simulink model "SecRwLtStZeroTrgtPosSelc"  (R2018b)
settings: Solver=FixedStepDiscrete  StartTime=0.0  StopTime=10.0  RelTol=1e-3
undefined symbols (not defined in the file or in its folder): KeSMSw6SAcsEntrySecRwLtStCushnFrtUpwdDnwdPos_Val, KeSMSw6SAcsEntrySecRwLtStCushnFrtUpwdDnwdPosMax_Val, KeSMSw6SAcsEntrySecRwLtStCushnFrtUpwdDnwdPosMin_Val, KeSMSw6SAcsMd56SecRwLtStCushnFrtUpwdDnwdPos_Val, KeSMSw6SAcsMd56SecRwLtStCushnFrtUpwdDnwdPosMax_Val, KeSMSw6SAcsMd56SecRwLtStCushnFrtUpwdDnwdPosMin_Val, KeSMSw6SRecoveryMdSecRwLtStCushnFrtUpwdDnwdPos_Val, KeSMSw6SRecoveryMdSecRwLtStCushnFrtUpwdDnwdPosMax_Val, KeSMSw6SRecoveryMdSecRwLtStCushnFrtUpwdDnwdPosMin_Val, KeSMSwAcsEntrySecRwLtStCushnFrtIUpwdDnwdPos_Val, KeSMSwAcsEntrySecRwLtStCushnFrtIUpwdDnwdPosMax_Val, KeSMSwAcsEntrySecRwLtStCushnFrtIUpwdDnwdPosMin_Val, KeSMSwAcsMd56SecRwLtStCushnFrtUpwdDnwdPos_Val, KeSMSwAcsMd56SecRwLtStCushnFrtUpwdDnwdPosMax_Val, KeSMSwAcsMd56SecRwLtStCushnFrtUpwdDnwdPosMin_Val, KeSMSwAcsMd8SecRwLtStCushnFrtUpwdDnwdPos_Val, KeSMSwAcsMd8SecRwLtStCushnFrtUpwdDnwdPosMax_Val, KeSMSwAcsMd8SecRwLtStCushnFrtUpwdDnwdPosMin_Val, KeSMSwRecoveryMdSecRwLtStCushnFrtUpwdDnwdPos_Val, KeSMSwRecoveryMdSecRwLtStCushnFrtUpwdDnwdPosMax_Val, KeSMSwRecoveryMdSecRwLtStCushnFrtUpwdDnwdPosMin_Val, KeSMSwSecRwLtStZeroEnTrig5576sBitMask_Val, KeSMSwSecRwLtStZeroEnTrig557BitMask_Val
libraries: TrgtPosSelcLib x5
settings Model: Creator=sn2xws  LastModifiedBy=sn2xws
settings Model: ModifiedHistory=|
  | 2024.7.8 V3.0.0 557模式流程V1.9
  | 2024.8.14 V3.0.1增加6s版bitmask标定
  | 2024.9.5 V3.0.2 增加Md56
  | 2024.9.16 V3.0.3 Md8 6s目标位置信号未连接到正确值（4095）
  | 2024.9.26 V3.0.4 只计算一次的目标位置创建static变量，避免丢失
settings DataIOCC: SaveFormat=StructureWithTime
settings OptimizationCC: DefaultParameterBehavior=Inlined  EnhancedBackFolding=on  PassReuseOutputArgsAs=Individual arguments  ZeroExternalMemoryAtStartup=off  ZeroInternalMemoryAtStartup=off  OptimizeBlockOrder=speed  DifferentSizesBufferReuse=on  OptimizationCustomize=off
settings DebuggingCC: ParameterTunabilityLossMsg=error
settings SFSimCC: MATLABDynamicMemAlloc=off
settings RTWCC: SystemTargetFile=autosar.tlc  GenCodeOnly=on  TemplateMakefile=ert_default_tmf  Description=AUTOSAR  GenerateReport=on  IncludeHyperlinkInReport=on  LaunchReport=on  GenerateTraceInfo=on  GenerateTraceReport=on  GenerateTraceReportSl=on  GenerateTraceReportSf=on  GenerateTraceReportEml=on
settings CodeAppCC: ForceParamTrailComments=on  IgnoreCustomStorageClasses=off  OperatorAnnotations=on  SimulinkDataObjDesc=on  SFDataObjDesc=on  InsertBlockDesc=on
settings STFCustomTargetCC: TargetLangStandard=C99 (ISO)  MultiwordLength=256  ParMdlRefBuildCompliant=on  CompOptLevelCompliant=on  IncludeMdlTerminateFcn=off  CombineOutputUpdateFcns=on  SuppressErrorStatus=on  ERTCustomFileBanners=on  SupportNonFinite=off  SupportComplex=off  SupportContinuousTime=off  SupportNonInlinedSFcns=off  RemoveResetFunc=on  MATLABClassNameForMDSCustomization=Simulink.SoftwareTarget.ERTCustomization  AutosarCompliant=on  UseToolchainInfoCompliant=on  LookupTableObjectStructAxisOrder=2,1,3,4,...  LUTObjectStructOrderEvenSpacing=Size,Table,Breakpoints  SystemTargetFile=autosar.tlc
settings ERTTargetCC: TargetLangStandard=C99 (ISO)  ConcurrentExecutionCompliant=off  IncludeMdlTerminateFcn=off  SuppressErrorStatus=on  SupportNonFinite=off  SupportComplex=off  ModelStepFunctionPrototypeControlCompliant=off  CPPClassGenCompliant=off  AutosarCompliant=on  LookupTableObjectStructAxisOrder=2,1,3,4,...  LUTObjectStructOrderEvenSpacing=Size,Table,Breakpoints  InlinedParameterPlacement=NonHierarchical  ERTCustomFileTemplate=example_file_process.tlc  ERTFilePackagingFormat=Compact

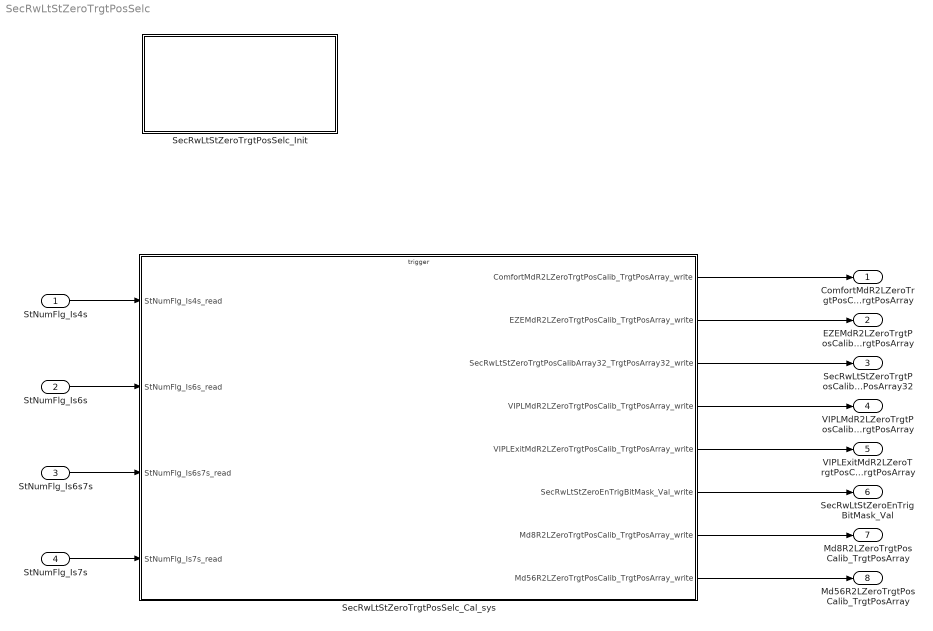
== system SecRwLtStZeroTrgtPosSelc ==
  StNumFlg_Is4s : Inport  OutDataTypeStr=boolean  PortDimensions=1
  StNumFlg_Is6s : Inport  Port=2  OutDataTypeStr=boolean  PortDimensions=1
  StNumFlg_Is6s7s : Inport  Port=3  OutDataTypeStr=boolean  PortDimensions=1
  StNumFlg_Is7s : Inport  Port=4  OutDataTypeStr=boolean  PortDimensions=1
  SecRwLtStZeroTrgtPosSelc_Cal_sys : Subsystem
  SecRwLtStZeroTrgtPosSelc_Init : Subsystem
  ComfortMdR2LZeroTrgtPosCalib_TrgtPosArray : Outport  Description=|  OutDataTypeStr=uint16  PortDimensions=3
      | 0:Pos
      | 1:Max
      | 2:Min
  EZEMdR2LZeroTrgtPosCalib_TrgtPosArray : Outport  Description=|  Port=2  OutDataTypeStr=uint16  PortDimensions=3
      | 0:Pos
      | 1:Max
      | 2:Min
  SecRwLtStZeroTrgtPosCalibArray32_TrgtPosArray32 : Outport  Description=|  Port=3  OutDataTypeStr=uint16  PortDimensions=96
      | 0:Pos
      | 1:Max
      | 2:Min
  VIPLMdR2LZeroTrgtPosCalib_TrgtPosArray : Outport  Description=|  Port=4  OutDataTypeStr=uint16  PortDimensions=3
      | 0:Pos
      | 1:Max
      | 2:Min
  VIPLExitMdR2LZeroTrgtPosCalib_TrgtPosArray : Outport  Description=|  Port=5  OutDataTypeStr=uint16  PortDimensions=3
      | 0:Pos
      | 1:Max
      | 2:Min
  SecRwLtStZeroEnTrigBitMask_Val : Outport  Port=6  OutDataTypeStr=uint32  PortDimensions=1
  Md8R2LZeroTrgtPosCalib_TrgtPosArray : Outport  Description=|  Port=7  OutDataTypeStr=uint16  PortDimensions=3
      | 0:Pos
      | 1:Max
      | 2:Min
  Md56R2LZeroTrgtPosCalib_TrgtPosArray : Outport  Description=|  Port=8  OutDataTypeStr=uint16  PortDimensions=3
      | 0:Pos
      | 1:Max
      | 2:Min
  wires:
  StNumFlg_Is4s/1 -> SecRwLtStZeroTrgtPosSelc_Cal_sys/1(StNumFlg_Is4s_read)
  StNumFlg_Is6s/1 -> SecRwLtStZeroTrgtPosSelc_Cal_sys/2(StNumFlg_Is6s_read)
  StNumFlg_Is6s7s/1 -> SecRwLtStZeroTrgtPosSelc_Cal_sys/3(StNumFlg_Is6s7s_read)
  StNumFlg_Is7s/1 -> SecRwLtStZeroTrgtPosSelc_Cal_sys/4(StNumFlg_Is7s_read)
  SecRwLtStZeroTrgtPosSelc_Cal_sys/1(ComfortMdR2LZeroTrgtPosCalib_TrgtPosArray_write) -> ComfortMdR2LZeroTrgtPosCalib_TrgtPosArray/1
  SecRwLtStZeroTrgtPosSelc_Cal_sys/2(EZEMdR2LZeroTrgtPosCalib_TrgtPosArray_write) -> EZEMdR2LZeroTrgtPosCalib_TrgtPosArray/1
  SecRwLtStZeroTrgtPosSelc_Cal_sys/3(SecRwLtStZeroTrgtPosCalibArray32_TrgtPosArray32_write) -> SecRwLtStZeroTrgtPosCalibArray32_TrgtPosArray32/1
  SecRwLtStZeroTrgtPosSelc_Cal_sys/4(VIPLMdR2LZeroTrgtPosCalib_TrgtPosArray_write) -> VIPLMdR2LZeroTrgtPosCalib_TrgtPosArray/1
  SecRwLtStZeroTrgtPosSelc_Cal_sys/5(VIPLExitMdR2LZeroTrgtPosCalib_TrgtPosArray_write) -> VIPLExitMdR2LZeroTrgtPosCalib_TrgtPosArray/1
  SecRwLtStZeroTrgtPosSelc_Cal_sys/6(SecRwLtStZeroEnTrigBitMask_Val_write) -> SecRwLtStZeroEnTrigBitMask_Val/1
  SecRwLtStZeroTrgtPosSelc_Cal_sys/7(Md8R2LZeroTrgtPosCalib_TrgtPosArray_write) -> Md8R2LZeroTrgtPosCalib_TrgtPosArray/1
  SecRwLtStZeroTrgtPosSelc_Cal_sys/8(Md56R2LZeroTrgtPosCalib_TrgtPosArray_write) -> Md56R2LZeroTrgtPosCalib_TrgtPosArray/1

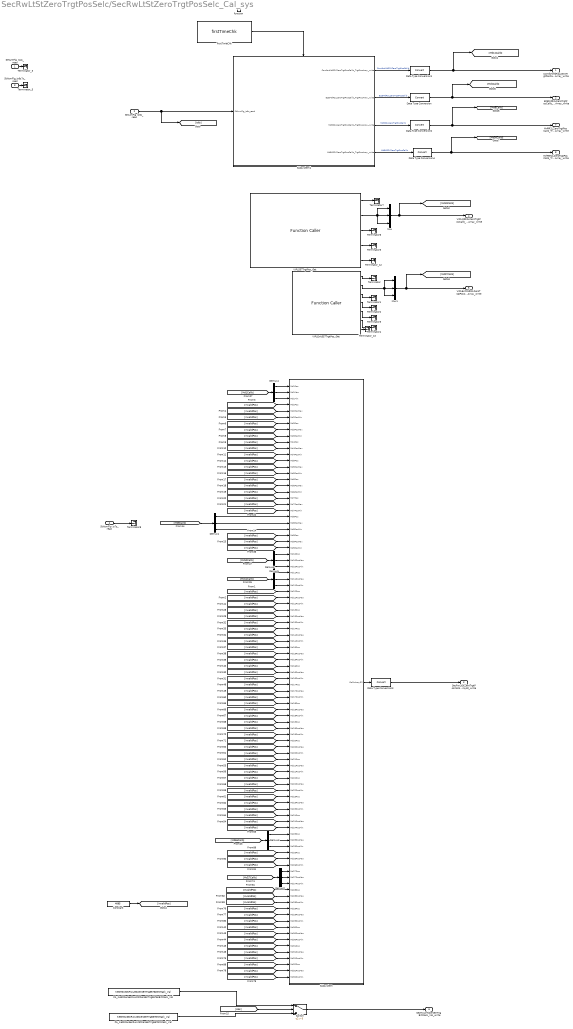
== system SecRwLtStZeroTrgtPosSelc/SecRwLtStZeroTrgtPosSelc_Cal_sys ==
  StNumFlg_Is4s_read : Inport
  StNumFlg_Is6s_read : Inport  Port=2
  StNumFlg_Is6s7s_read : Inport  Port=3
  StNumFlg_Is7s_read : Inport  Port=4
  function : TriggerPort  TriggerType=function-call  IsSimulinkFunction=on  FunctionName=SecRwLtStZeroTrgtPosSelc_Cal  VariantControl=(inherit)
  Constant : Constant  Value=4095  OutDataTypeStr=uint16
  Data Type Conversion{,1..4} (5 alike) : DataTypeConversion
  Demux{1..6} (6 alike) : Demux  Outputs=3
  Mux : Mux  Inputs=3
  Mux1 : Mux  Inputs=3
  PA_KeSMSwSecRwLtStZeroEnTrig5576sBitMask_Val : Constant  Value=KeSMSwSecRwLtStZeroEnTrig5576sBitMask_Val
  PA_KeSMSwSecRwLtStZeroEnTrig557BitMask_Val : Constant  Value=KeSMSwSecRwLtStZeroEnTrig557BitMask_Val
  Subsystem : Subsystem
  Subsystem1 : Subsystem
  Switch : Switch  Criteria=u2 > Threshold
  Terminator{,1..8} (9 alike) : Terminator
  Terminator_{3,5,12..13} (4 alike) : Terminator
  VIPL557TrgtPos_Get : FunctionCaller  FunctionPrototype=[SecRwLtStBkReclnTrgtPos,SecRwLtStZeroTrgtPos,SecRwLtStLgrstUpwdDnwdTrgtPos,SecRwLtStLgrstInwdOtwdTrgtPos,SecRwLtStFwdBkwdTrgtPos] = VIPL557TrgtPos_Get()  OutputArgumentSpecifications=uint16(1), uint16(1), uint16(1), uint16(1), uint16(1)
  VIPLExit557TrgtPos_Get : FunctionCaller  FunctionPrototype=[SecRwLtStBkReclnTrgtPos,SecRwLtStZeroTrgtPos,SecRwLtStLgrstUpwdDnwdTrgtPos,SecRwLtStLgrstInwdOtwdTrgtPos,ThdRwLtStBkReclnTrgtPos,ThdRwLtStFwdBkwdTrgtPos,SecRwLtStFwdBkwdTrgtPos] = VIPLExit557TrgtPos_Get()  OutputArgumentSpecifications=uint16(1), uint16(1), uint16(1), uint16(1), uint16(1), uint16(1), uint16(1)
  firstTimeChk : TrgtPosSelcLib/firstTimeChk  SystemSampleTime=-1
  ComfortMdR2LZeroTrgtPosCalib_TrgtPosArray_write : Outport
      settings: EnsureOutportIsVirtual=on
  EZEMdR2LZeroTrgtPosCalib_TrgtPosArray_write : Outport  Port=2
      settings: EnsureOutportIsVirtual=on
  SecRwLtStZeroTrgtPosCalibArray32_TrgtPosArray32_write : Outport  Port=3
      settings: EnsureOutportIsVirtual=on
  VIPLMdR2LZeroTrgtPosCalib_TrgtPosArray_write : Outport  Port=4
      settings: EnsureOutportIsVirtual=on
  VIPLExitMdR2LZeroTrgtPosCalib_TrgtPosArray_write : Outport  Port=5
      settings: EnsureOutportIsVirtual=on
  SecRwLtStZeroEnTrigBitMask_Val_write : Outport  Port=6
      settings: EnsureOutportIsVirtual=on
  Md8R2LZeroTrgtPosCalib_TrgtPosArray_write : Outport  Port=7
      settings: EnsureOutportIsVirtual=on
  Md56R2LZeroTrgtPosCalib_TrgtPosArray_write : Outport  Port=8
      settings: EnsureOutportIsVirtual=on
  wires:
  StNumFlg_Is4s_read/1 -> Terminator_3/1
  StNumFlg_Is6s7s_read/1 -> Terminator_5/1
  Mux/1 -> [Md10Calib], VIPLMdR2LZeroTrgtPosCalib_TrgtPosArray_write/1
  VIPLExit557TrgtPos_Get/2 -> Mux1/3, Mux1/1, Mux1/2
  Mux1/1 -> [Md27Calib], VIPLExitMdR2LZeroTrgtPosCalib_TrgtPosArray_write/1
  VIPLExit557TrgtPos_Get/1 -> Terminator/1
  VIPLExit557TrgtPos_Get/3 -> Terminator1/1
  VIPLExit557TrgtPos_Get/4 -> Terminator2/1
  VIPLExit557TrgtPos_Get/5 -> Terminator3/1
  VIPLExit557TrgtPos_Get/6 -> Terminator4/1
  VIPL557TrgtPos_Get/4 -> Terminator5/1
  VIPL557TrgtPos_Get/3 -> Terminator6/1
  VIPL557TrgtPos_Get/1 -> Terminator7/1
  VIPL557TrgtPos_Get/2 -> Mux/3, Mux/1, Mux/2
  Data Type Conversion3/1 -> SecRwLtStZeroTrgtPosCalibArray32_TrgtPosArray32_write/1
  Demux1/3 -> Subsystem/24(Md8PosMin)
  [invalidPos] -> Subsystem/85(Md29Pos)
  [invalidPos] -> Subsystem/10(Md4Pos)
  [invalidPos] -> Subsystem/17(Md6PosMax)
  [invalidPos] -> Subsystem/50(Md17PosMax)
  [invalidPos] -> Subsystem/77(Md26PosMax)
  Demux1/1 -> Subsystem/22(Md8Pos)
  [invalidPos] -> Subsystem/9(Md3PosMin)
  [invalidPos] -> Subsystem/76(Md26Pos)
  [invalidPos] -> Subsystem/25(Md9Pos)
  [invalidPos] -> Subsystem/46(Md16Pos)
  [invalidPos] -> Subsystem/72(Md24PosMin)
  Demux5/3 -> Subsystem/30(Md10PosMin)
  [invalidPos] -> Subsystem/45(Md15PosMin)
  [invalidPos] -> Subsystem/20(Md7PosMax)
  [invalidPos] -> Subsystem/63(Md21PosMin)
  [invalidPos] -> Subsystem/58(Md20Pos)
  [invalidPos] -> Subsystem/53(Md18PosMax)
  Demux4/1 -> Subsystem/1(Md1Pos)
  [invalidPos] -> Subsystem/55(Md19Pos)
  [invalidPos] -> Subsystem/86(Md29PosMax)
  [invalidPos] -> Subsystem/68(Md23PosMax)
  [invalidPos] -> Subsystem/62(Md21PosMax)
  [invalidPos] -> Subsystem/14(Md5PosMax)
  [invalidPos] -> Subsystem/87(Md29PosMin)
  Demux1/2 -> Subsystem/23(Md8PosMax)
  [invalidPos] -> Subsystem/26(Md9PosMax)
  [invalidPos] -> Subsystem/94(Md32Pos)
  [invalidPos] -> Subsystem/54(Md18PosMin)
  [invalidPos] -> Subsystem/61(Md21Pos)
  [invalidPos] -> Subsystem/5(Md2PosMax)
  [invalidPos] -> Subsystem/13(Md5Pos)
  [invalidPos] -> Subsystem/96(Md32PosMin)
  [invalidPos] -> Subsystem/59(Md20PosMax)
  [invalidPos] -> Subsystem/78(Md26PosMin)
  [invalidPos] -> Subsystem/11(Md4PosMax)
  Demux3/1 -> Subsystem/73(Md25Pos)
  [invalidPos] -> Subsystem/66(Md22PosMin)
  [invalidPos] -> Subsystem/16(Md6Pos)
  Demux4/2 -> Subsystem/2(Md1Max)
  [invalidPos] -> Subsystem/70(Md24Pos)
  [invalidPos] -> Subsystem/44(Md15PosMax)
  [invalidPos] -> Subsystem/60(Md20PosMin)
  [invalidPos] -> Subsystem/64(Md22Pos)
  [invalidPos] -> Subsystem/51(Md17PosMin)
  [invalidPos] -> Subsystem/43(Md15Pos)
  [invalidPos] -> Subsystem/57(Md19PosMin)
  [invalidPos] -> Subsystem/18(Md6PosMin)
  [invalidPos] -> Subsystem/67(Md23Pos)
  [invalidPos] -> Subsystem/4(Md2Pos)
  [invalidPos] -> Subsystem/49(Md17Pos)
  [invalidPos] -> Subsystem/71(Md24PosMax)
  [invalidPos] -> Subsystem/65(Md22PosMax)
  [invalidPos] -> Subsystem/6(Md2PosMin)
  Demux3/3 -> Subsystem/75(Md25PosMin)
  [invalidPos] -> Subsystem/37(Md13Pos)
  [invalidPos] -> Subsystem/52(Md18Pos)
  Demux3/2 -> Subsystem/74(Md25PosMax)
  [invalidPos] -> Subsystem/27(Md9PosMin)
  [invalidPos] -> Subsystem/48(Md16PosMin)
  [invalidPos] -> Subsystem/41(Md14PosMax)
  Demux5/1 -> Subsystem/28(Md10Pos)
  [invalidPos] -> Subsystem/38(Md13PosMax)
  [invalidPos] -> Subsystem/47(Md16PosMax)
  [invalidPos] -> Subsystem/56(Md19PosMax)
  [invalidPos] -> Subsystem/39(Md13PosMin)
  [invalidPos] -> Subsystem/40(Md14Pos)
  Subsystem/1(CalibArray32) -> Data Type Conversion3/1
  [invalidPos] -> Subsystem/42(Md14PosMin)
  [invalidPos] -> Subsystem/21(Md7PosMin)
  [invalidPos] -> Subsystem/19(Md7Pos)
  [invalidPos] -> Subsystem/12(Md4PosMin)
  [invalidPos] -> Subsystem/69(Md23PosMin)
  [invalidPos] -> Subsystem/82(Md28Pos)
  [invalidPos] -> Subsystem/15(Md5PosMin)
  Demux4/3 -> Subsystem/3(Md1Min)
  [invalidPos] -> Subsystem/95(Md32PosMax)
  [invalidPos] -> Subsystem/8(Md3PosMax)
  [invalidPos] -> Subsystem/7(Md3Pos)
  Demux5/2 -> Subsystem/29(Md10PosMax)
  [Md1Calib] -> Demux4/1
  [Md10Calib] -> Demux5/1
  Demux6/1 -> Subsystem/31(Md11Pos)
  Demux6/2 -> Subsystem/32(Md11PosMax)
  Demux6/3 -> Subsystem/33(Md11PosMin)
  [Md11Calib] -> Demux6/1
  [invalidPos] -> Subsystem/34(Md12Pos)
  [invalidPos] -> Subsystem/35(Md12PosMax)
  [invalidPos] -> Subsystem/36(Md12PosMin)
  [Md27Calib] -> Demux2/1
  Demux2/1 -> Subsystem/79(Md27Pos)
  Demux2/2 -> Subsystem/80(Md27PosMax)
  Demux2/3 -> Subsystem/81(Md27PosMin)
  [invalidPos] -> Subsystem/83(Md28PosMax)
  [invalidPos] -> Subsystem/84(Md28PosMin)
  [invalidPos] -> Subsystem/88(Md30Pos)
  [invalidPos] -> Subsystem/89(Md30PosMax)
  [invalidPos] -> Subsystem/90(Md30PosMin)
  [invalidPos] -> Subsystem/91(Md31Pos)
  [invalidPos] -> Subsystem/92(Md31PosMax)
  [invalidPos] -> Subsystem/93(Md31PosMin)
  Constant/1 -> [invalidPos]
  VIPL557TrgtPos_Get/5 -> Terminator_12/1
  VIPLExit557TrgtPos_Get/7 -> Terminator_13/1
  [Md8Calib] -> Demux1/1
  StNumFlg_Is7s_read/1 -> Terminator8/1
  Switch/1 -> SecRwLtStZeroEnTrigBitMask_Val_write/1
  [Is6s] -> Switch/2
  PA_KeSMSwSecRwLtStZeroEnTrig5576sBitMask_Val/1 -> Switch/1
  PA_KeSMSwSecRwLtStZeroEnTrig557BitMask_Val/1 -> Switch/3
  firstTimeChk/1 -> Subsystem1/Enable
  StNumFlg_Is6s_read/1 -> [Is6s], Subsystem1/1(StNumFlg_Is6s_read)
  Subsystem1/4(Md56R2LZeroTrgtPosCalib_TrgtPosArray_write) -> Data Type Conversion4/1  "Md56R2LZeroTrgtPosCalib"
  Subsystem1/1(ComfortMdR2LZeroTrgtPosCalib_TrgtPosArray_write) -> Data Type Conversion1/1  "ComfortMdR2LZeroTrgtPosCalib"
  Subsystem1/2(EZEMdR2LZeroTrgtPosCalib_TrgtPosArray_write) -> Data Type Conversion/1  "EZEMdR2LZeroTrgtPosCalib"
  Subsystem1/3(Md8R2LZeroTrgtPosCalib_TrgtPosArray_write) -> Data Type Conversion2/1  "Md8R2LZeroTrgtPosCalib"
  [Md56Calib] -> Demux3/1
  Data Type Conversion1/1 -> [Md11Calib], ComfortMdR2LZeroTrgtPosCalib_TrgtPosArray_write/1
  Data Type Conversion/1 -> [Md1Calib], EZEMdR2LZeroTrgtPosCalib_TrgtPosArray_write/1
  Data Type Conversion2/1 -> [Md8Calib], Md8R2LZeroTrgtPosCalib_TrgtPosArray_write/1
  Data Type Conversion4/1 -> [Md56Calib], Md56R2LZeroTrgtPosCalib_TrgtPosArray_write/1

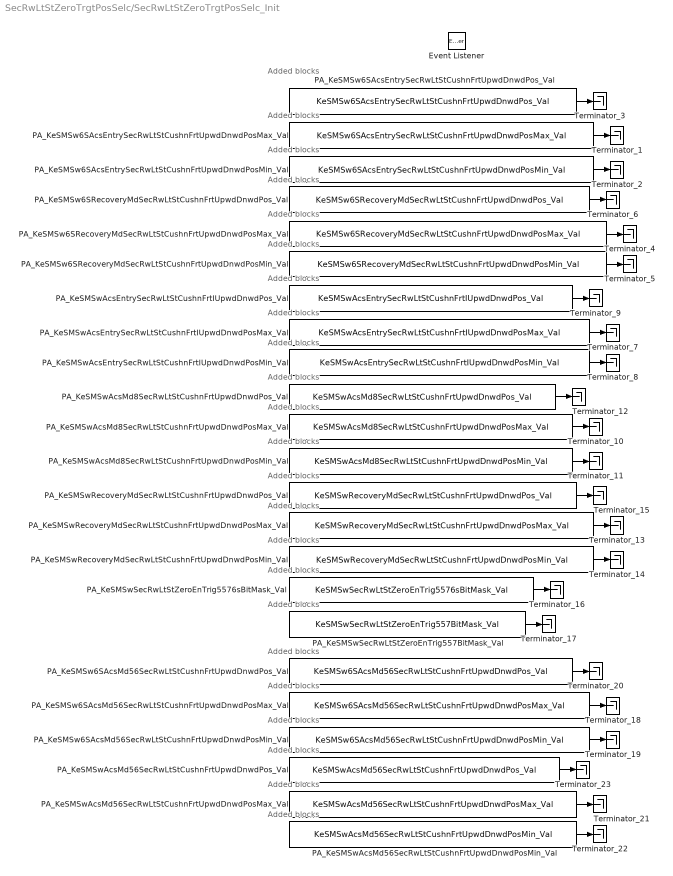
== system SecRwLtStZeroTrgtPosSelc/SecRwLtStZeroTrgtPosSelc_Init ==
  note: Added blocks
  note: Added blocks
  note: Added blocks
  note: Added blocks
  note: Added blocks
  note: Added blocks
  note: Added blocks
  note: Added blocks
  note: Added blocks
  note: Added blocks
  note: Added blocks
  note: Added blocks
  note: Added blocks
  note: Added blocks
  note: Added blocks
  note: Added blocks
  note: Added blocks
  note: Added blocks
  note: Added blocks
  note: Added blocks
  note: Added blocks
  note: Added blocks
  note: Added blocks
  Event Listener : EventListener  EventName=reset
  PA_KeSMSw6SAcsEntrySecRwLtStCushnFrtUpwdDnwdPosMax_Val : Constant  Value=KeSMSw6SAcsEntrySecRwLtStCushnFrtUpwdDnwdPosMax_Val
  PA_KeSMSw6SAcsEntrySecRwLtStCushnFrtUpwdDnwdPosMin_Val : Constant  Value=KeSMSw6SAcsEntrySecRwLtStCushnFrtUpwdDnwdPosMin_Val
  PA_KeSMSw6SAcsEntrySecRwLtStCushnFrtUpwdDnwdPos_Val : Constant  Value=KeSMSw6SAcsEntrySecRwLtStCushnFrtUpwdDnwdPos_Val
  PA_KeSMSw6SAcsMd56SecRwLtStCushnFrtUpwdDnwdPosMax_Val : Constant  Value=KeSMSw6SAcsMd56SecRwLtStCushnFrtUpwdDnwdPosMax_Val
  PA_KeSMSw6SAcsMd56SecRwLtStCushnFrtUpwdDnwdPosMin_Val : Constant  Value=KeSMSw6SAcsMd56SecRwLtStCushnFrtUpwdDnwdPosMin_Val
  PA_KeSMSw6SAcsMd56SecRwLtStCushnFrtUpwdDnwdPos_Val : Constant  Value=KeSMSw6SAcsMd56SecRwLtStCushnFrtUpwdDnwdPos_Val
  PA_KeSMSw6SRecoveryMdSecRwLtStCushnFrtUpwdDnwdPosMax_Val : Constant  Value=KeSMSw6SRecoveryMdSecRwLtStCushnFrtUpwdDnwdPosMax_Val
  PA_KeSMSw6SRecoveryMdSecRwLtStCushnFrtUpwdDnwdPosMin_Val : Constant  Value=KeSMSw6SRecoveryMdSecRwLtStCushnFrtUpwdDnwdPosMin_Val
  PA_KeSMSw6SRecoveryMdSecRwLtStCushnFrtUpwdDnwdPos_Val : Constant  Value=KeSMSw6SRecoveryMdSecRwLtStCushnFrtUpwdDnwdPos_Val
  PA_KeSMSwAcsEntrySecRwLtStCushnFrtIUpwdDnwdPosMax_Val : Constant  Value=KeSMSwAcsEntrySecRwLtStCushnFrtIUpwdDnwdPosMax_Val
  PA_KeSMSwAcsEntrySecRwLtStCushnFrtIUpwdDnwdPosMin_Val : Constant  Value=KeSMSwAcsEntrySecRwLtStCushnFrtIUpwdDnwdPosMin_Val
  PA_KeSMSwAcsEntrySecRwLtStCushnFrtIUpwdDnwdPos_Val : Constant  Value=KeSMSwAcsEntrySecRwLtStCushnFrtIUpwdDnwdPos_Val
  PA_KeSMSwAcsMd56SecRwLtStCushnFrtUpwdDnwdPosMax_Val : Constant  Value=KeSMSwAcsMd56SecRwLtStCushnFrtUpwdDnwdPosMax_Val
  PA_KeSMSwAcsMd56SecRwLtStCushnFrtUpwdDnwdPosMin_Val : Constant  Value=KeSMSwAcsMd56SecRwLtStCushnFrtUpwdDnwdPosMin_Val
  PA_KeSMSwAcsMd56SecRwLtStCushnFrtUpwdDnwdPos_Val : Constant  Value=KeSMSwAcsMd56SecRwLtStCushnFrtUpwdDnwdPos_Val
  PA_KeSMSwAcsMd8SecRwLtStCushnFrtUpwdDnwdPosMax_Val : Constant  Value=KeSMSwAcsMd8SecRwLtStCushnFrtUpwdDnwdPosMax_Val
  PA_KeSMSwAcsMd8SecRwLtStCushnFrtUpwdDnwdPosMin_Val : Constant  Value=KeSMSwAcsMd8SecRwLtStCushnFrtUpwdDnwdPosMin_Val
  PA_KeSMSwAcsMd8SecRwLtStCushnFrtUpwdDnwdPos_Val : Constant  Value=KeSMSwAcsMd8SecRwLtStCushnFrtUpwdDnwdPos_Val
  PA_KeSMSwRecoveryMdSecRwLtStCushnFrtUpwdDnwdPosMax_Val : Constant  Value=KeSMSwRecoveryMdSecRwLtStCushnFrtUpwdDnwdPosMax_Val
  PA_KeSMSwRecoveryMdSecRwLtStCushnFrtUpwdDnwdPosMin_Val : Constant  Value=KeSMSwRecoveryMdSecRwLtStCushnFrtUpwdDnwdPosMin_Val
  PA_KeSMSwRecoveryMdSecRwLtStCushnFrtUpwdDnwdPos_Val : Constant  Value=KeSMSwRecoveryMdSecRwLtStCushnFrtUpwdDnwdPos_Val
  PA_KeSMSwSecRwLtStZeroEnTrig5576sBitMask_Val : Constant  Value=KeSMSwSecRwLtStZeroEnTrig5576sBitMask_Val
  PA_KeSMSwSecRwLtStZeroEnTrig557BitMask_Val : Constant  Value=KeSMSwSecRwLtStZeroEnTrig557BitMask_Val
  Terminator_{1..23} (23 alike) : Terminator
  wires:
  PA_KeSMSw6SAcsEntrySecRwLtStCushnFrtUpwdDnwdPosMax_Val/1 -> Terminator_1/1
  PA_KeSMSw6SAcsEntrySecRwLtStCushnFrtUpwdDnwdPosMin_Val/1 -> Terminator_2/1
  PA_KeSMSw6SAcsEntrySecRwLtStCushnFrtUpwdDnwdPos_Val/1 -> Terminator_3/1
  PA_KeSMSw6SRecoveryMdSecRwLtStCushnFrtUpwdDnwdPosMax_Val/1 -> Terminator_4/1
  PA_KeSMSw6SRecoveryMdSecRwLtStCushnFrtUpwdDnwdPosMin_Val/1 -> Terminator_5/1
  PA_KeSMSw6SRecoveryMdSecRwLtStCushnFrtUpwdDnwdPos_Val/1 -> Terminator_6/1
  PA_KeSMSwAcsEntrySecRwLtStCushnFrtIUpwdDnwdPosMax_Val/1 -> Terminator_7/1
  PA_KeSMSwAcsEntrySecRwLtStCushnFrtIUpwdDnwdPosMin_Val/1 -> Terminator_8/1
  PA_KeSMSwAcsEntrySecRwLtStCushnFrtIUpwdDnwdPos_Val/1 -> Terminator_9/1
  PA_KeSMSwAcsMd8SecRwLtStCushnFrtUpwdDnwdPosMax_Val/1 -> Terminator_10/1
  PA_KeSMSwAcsMd8SecRwLtStCushnFrtUpwdDnwdPosMin_Val/1 -> Terminator_11/1
  PA_KeSMSwAcsMd8SecRwLtStCushnFrtUpwdDnwdPos_Val/1 -> Terminator_12/1
  PA_KeSMSwRecoveryMdSecRwLtStCushnFrtUpwdDnwdPosMax_Val/1 -> Terminator_13/1
  PA_KeSMSwRecoveryMdSecRwLtStCushnFrtUpwdDnwdPosMin_Val/1 -> Terminator_14/1
  PA_KeSMSwRecoveryMdSecRwLtStCushnFrtUpwdDnwdPos_Val/1 -> Terminator_15/1
  PA_KeSMSwSecRwLtStZeroEnTrig5576sBitMask_Val/1 -> Terminator_16/1
  PA_KeSMSwSecRwLtStZeroEnTrig557BitMask_Val/1 -> Terminator_17/1
  PA_KeSMSw6SAcsMd56SecRwLtStCushnFrtUpwdDnwdPosMax_Val/1 -> Terminator_18/1
  PA_KeSMSw6SAcsMd56SecRwLtStCushnFrtUpwdDnwdPosMin_Val/1 -> Terminator_19/1
  PA_KeSMSw6SAcsMd56SecRwLtStCushnFrtUpwdDnwdPos_Val/1 -> Terminator_20/1
  PA_KeSMSwAcsMd56SecRwLtStCushnFrtUpwdDnwdPosMax_Val/1 -> Terminator_21/1
  PA_KeSMSwAcsMd56SecRwLtStCushnFrtUpwdDnwdPosMin_Val/1 -> Terminator_22/1
  PA_KeSMSwAcsMd56SecRwLtStCushnFrtUpwdDnwdPos_Val/1 -> Terminator_23/1

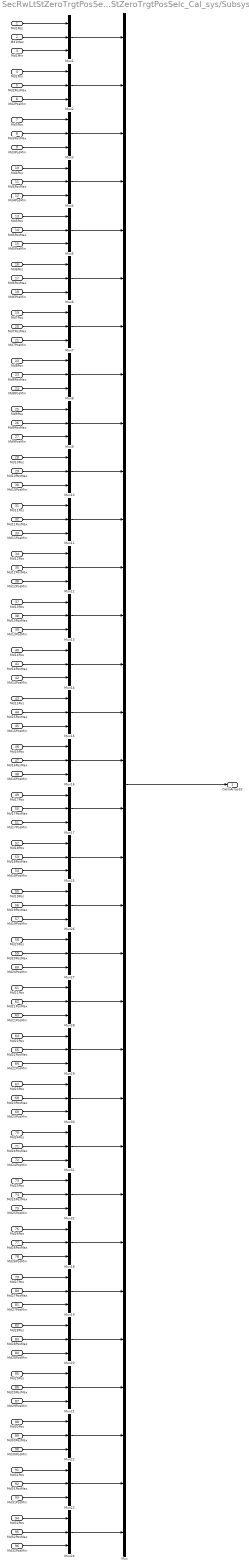
== system SecRwLtStZeroTrgtPosSelc/SecRwLtStZeroTrgtPosSelc_Cal_sys/Subsystem ==
  Md1Pos : Inport
  Md1Max : Inport  Port=2
  Md1Min : Inport  Port=3
  Md2Pos : Inport  Port=4
  Md2PosMax : Inport  Port=5
  Md2PosMin : Inport  Port=6
  Md3Pos : Inport  Port=7
  Md3PosMax : Inport  Port=8
  Md3PosMin : Inport  Port=9
  Md4Pos : Inport  Port=10
  Md4PosMax : Inport  Port=11
  Md4PosMin : Inport  Port=12
  Md5Pos : Inport  Port=13
  Md5PosMax : Inport  Port=14
  Md5PosMin : Inport  Port=15
  Md6Pos : Inport  Port=16
  Md6PosMax : Inport  Port=17
  Md6PosMin : Inport  Port=18
  Md7Pos : Inport  Port=19
  Md7PosMax : Inport  Port=20
  Md7PosMin : Inport  Port=21
  Md8Pos : Inport  Port=22
  Md8PosMax : Inport  Port=23
  Md8PosMin : Inport  Port=24
  Md9Pos : Inport  Port=25
  Md9PosMax : Inport  Port=26
  Md9PosMin : Inport  Port=27
  Md10Pos : Inport  Port=28
  Md10PosMax : Inport  Port=29
  Md10PosMin : Inport  Port=30
  Md11Pos : Inport  Port=31
  Md11PosMax : Inport  Port=32
  Md11PosMin : Inport  Port=33
  Md12Pos : Inport  Port=34
  Md12PosMax : Inport  Port=35
  Md12PosMin : Inport  Port=36
  Md13Pos : Inport  Port=37
  Md13PosMax : Inport  Port=38
  Md13PosMin : Inport  Port=39
  Md14Pos : Inport  Port=40
  Md14PosMax : Inport  Port=41
  Md14PosMin : Inport  Port=42
  Md15Pos : Inport  Port=43
  Md15PosMax : Inport  Port=44
  Md15PosMin : Inport  Port=45
  Md16Pos : Inport  Port=46
  Md16PosMax : Inport  Port=47
  Md16PosMin : Inport  Port=48
  Md17Pos : Inport  Port=49
  Md17PosMax : Inport  Port=50
  Md17PosMin : Inport  Port=51
  Md18Pos : Inport  Port=52
  Md18PosMax : Inport  Port=53
  Md18PosMin : Inport  Port=54
  Md19Pos : Inport  Port=55
  Md19PosMax : Inport  Port=56
  Md19PosMin : Inport  Port=57
  Md20Pos : Inport  Port=58
  Md20PosMax : Inport  Port=59
  Md20PosMin : Inport  Port=60
  Md21Pos : Inport  Port=61
  Md21PosMax : Inport  Port=62
  Md21PosMin : Inport  Port=63
  Md22Pos : Inport  Port=64
  Md22PosMax : Inport  Port=65
  Md22PosMin : Inport  Port=66
  Md23Pos : Inport  Port=67
  Md23PosMax : Inport  Port=68
  Md23PosMin : Inport  Port=69
  Md24Pos : Inport  Port=70
  Md24PosMax : Inport  Port=71
  Md24PosMin : Inport  Port=72
  Md25Pos : Inport  Port=73
  Md25PosMax : Inport  Port=74
  Md25PosMin : Inport  Port=75
  Md26Pos : Inport  Port=76
  Md26PosMax : Inport  Port=77
  Md26PosMin : Inport  Port=78
  Md27Pos : Inport  Port=79
  Md27PosMax : Inport  Port=80
  Md27PosMin : Inport  Port=81
  Md28Pos : Inport  Port=82
  Md28PosMax : Inport  Port=83
  Md28PosMin : Inport  Port=84
  Md29Pos : Inport  Port=85
  Md29PosMax : Inport  Port=86
  Md29PosMin : Inport  Port=87
  Md30Pos : Inport  Port=88
  Md30PosMax : Inport  Port=89
  Md30PosMin : Inport  Port=90
  Md31Pos : Inport  Port=91
  Md31PosMax : Inport  Port=92
  Md31PosMin : Inport  Port=93
  Md32Pos : Inport  Port=94
  Md32PosMax : Inport  Port=95
  Md32PosMin : Inport  Port=96
  Mux : Mux  Inputs=32
  Mux{1..32} (32 alike) : Mux  Inputs=3
  CalibArray32 : Outport
  wires:
  Md22PosMax/1 -> Mux29/2
  Md3PosMin/1 -> Mux3/3
  Mux13/1 -> Mux/13
  Md13Pos/1 -> Mux13/1
  Mux30/1 -> Mux/23
  Md2PosMax/1 -> Mux2/2
  Md12PosMin/1 -> Mux12/3
  Md15PosMax/1 -> Mux15/2
  Md17Pos/1 -> Mux17/1
  Mux20/1 -> Mux/28
  Mux27/1 -> Mux/20
  Mux11/1 -> Mux/11
  Mux31/1 -> Mux/24
  Mux24/1 -> Mux/32
  Md8PosMin/1 -> Mux8/3
  Mux7/1 -> Mux/7
  Md20Pos/1 -> Mux27/1
  Mux6/1 -> Mux/6
  Md2PosMin/1 -> Mux2/3
  Md2Pos/1 -> Mux2/1
  Md5Pos/1 -> Mux5/1
  Md4PosMax/1 -> Mux4/2
  Mux25/1 -> Mux/18
  Md5PosMin/1 -> Mux5/3
  Md16PosMin/1 -> Mux16/3
  Md12PosMax/1 -> Mux12/2
  Mux32/1 -> Mux/25
  Md15PosMin/1 -> Mux15/3
  Mux15/1 -> Mux/15
  Mux16/1 -> Mux/16
  Mux21/1 -> Mux/29
  Md27PosMax/1 -> Mux19/2
  Md28Pos/1 -> Mux20/1
  Md13PosMin/1 -> Mux13/3
  Mux29/1 -> Mux/22
  Md8Pos/1 -> Mux8/1
  Mux23/1 -> Mux/31
  Mux22/1 -> Mux/30
  Mux12/1 -> Mux/12
  Md24Pos/1 -> Mux31/1
  Mux9/1 -> Mux/9
  Mux8/1 -> Mux/8
  Md9Pos/1 -> Mux9/1
  Mux3/1 -> Mux/3
  Md6PosMin/1 -> Mux6/3
  Mux17/1 -> Mux/17
  Md6Pos/1 -> Mux6/1
  Mux14/1 -> Mux/14
  Mux1/1 -> Mux/1
  Md10Pos/1 -> Mux10/1
  Md9PosMax/1 -> Mux9/2
  Mux26/1 -> Mux/19
  Mux18/1 -> Mux/26
  Mux28/1 -> Mux/21
  Mux2/1 -> Mux/2
  Mux19/1 -> Mux/27
  Mux10/1 -> Mux/10
  Mux5/1 -> Mux/5
  Md23PosMin/1 -> Mux30/3
  Md4PosMin/1 -> Mux4/3
  Md7PosMin/1 -> Mux7/3
  Md4Pos/1 -> Mux4/1
  Mux4/1 -> Mux/4
  Md13PosMax/1 -> Mux13/2
  Md6PosMax/1 -> Mux6/2
  Md5PosMax/1 -> Mux5/2
  Md14PosMax/1 -> Mux14/2
  Md14PosMin/1 -> Mux14/3
  Md23PosMax/1 -> Mux30/2
  Md1Min/1 -> Mux1/3
  Md8PosMax/1 -> Mux8/2
  Md23Pos/1 -> Mux30/1
  Md1Pos/1 -> Mux1/1
  Md1Max/1 -> Mux1/2
  Md9PosMin/1 -> Mux9/3
  Md7PosMax/1 -> Mux7/2
  Md20PosMin/1 -> Mux27/3
  Md7Pos/1 -> Mux7/1
  Md10PosMax/1 -> Mux10/2
  Md10PosMin/1 -> Mux10/3
  Md15Pos/1 -> Mux15/1
  Md30PosMax/1 -> Mux22/2
  Md11PosMax/1 -> Mux11/2
  Md12Pos/1 -> Mux12/1
  Md11PosMin/1 -> Mux11/3
  Md11Pos/1 -> Mux11/1
  Md14Pos/1 -> Mux14/1
  Md16Pos/1 -> Mux16/1
  Md24PosMin/1 -> Mux31/3
  Md16PosMax/1 -> Mux16/2
  Md32PosMin/1 -> Mux24/3
  Md27Pos/1 -> Mux19/1
  Md32PosMax/1 -> Mux24/2
  Md18Pos/1 -> Mux25/1
  Md19Pos/1 -> Mux26/1
  Md19PosMax/1 -> Mux26/2
  Md21Pos/1 -> Mux28/1
  Md27PosMin/1 -> Mux19/3
  Md26PosMax/1 -> Mux18/2
  Md26PosMin/1 -> Mux18/3
  Md31Pos/1 -> Mux23/1
  Md25Pos/1 -> Mux32/1
  Md28PosMin/1 -> Mux20/3
  Md25PosMin/1 -> Mux32/3
  Md25PosMax/1 -> Mux32/2
  Md17PosMin/1 -> Mux17/3
  Md32Pos/1 -> Mux24/1
  Md24PosMax/1 -> Mux31/2
  Md18PosMax/1 -> Mux25/2
  Md21PosMin/1 -> Mux28/3
  Md30PosMin/1 -> Mux22/3
  Md21PosMax/1 -> Mux28/2
  Md22Pos/1 -> Mux29/1
  Md18PosMin/1 -> Mux25/3
  Md26Pos/1 -> Mux18/1
  Md20PosMax/1 -> Mux27/2
  Md31PosMin/1 -> Mux23/3
  Md29Pos/1 -> Mux21/1
  Md19PosMin/1 -> Mux26/3
  Md29PosMin/1 -> Mux21/3
  Md30Pos/1 -> Mux22/1
  Md17PosMax/1 -> Mux17/2
  Md28PosMax/1 -> Mux20/2
  Md22PosMin/1 -> Mux29/3
  Md31PosMax/1 -> Mux23/2
  Md29PosMax/1 -> Mux21/2
  Mux/1 -> CalibArray32/1
  Md3Pos/1 -> Mux3/1
  Md3PosMax/1 -> Mux3/2

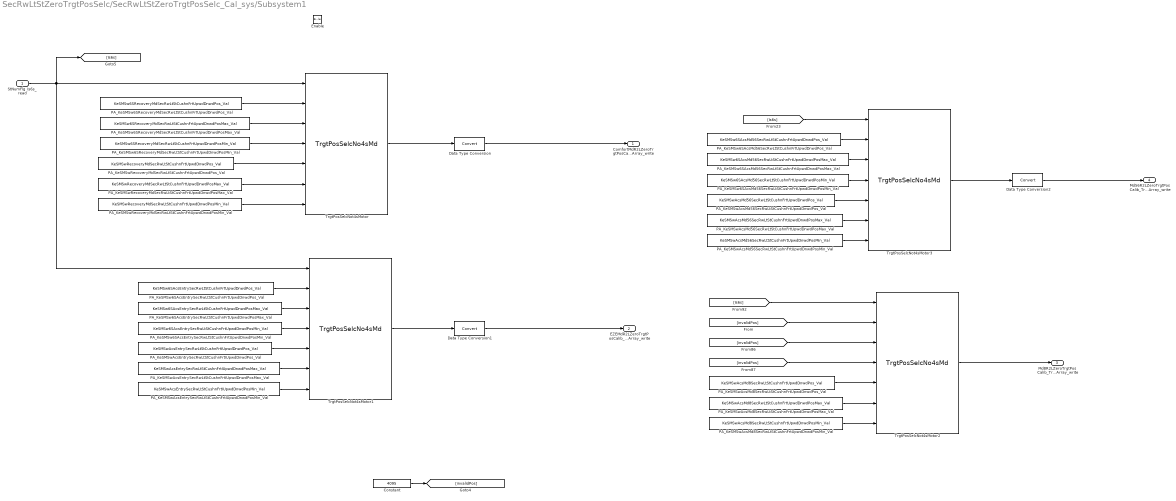
== system SecRwLtStZeroTrgtPosSelc/SecRwLtStZeroTrgtPosSelc_Cal_sys/Subsystem1 ==
  StNumFlg_Is6s_read : Inport
  Enable : EnablePort
  Constant : Constant  Value=4095  OutDataTypeStr=uint16
  Data Type Conversion : DataTypeConversion
  Data Type Conversion1 : DataTypeConversion
  Data Type Conversion2 : DataTypeConversion
  PA_KeSMSw6SAcsEntrySecRwLtStCushnFrtUpwdDnwdPosMax_Val : Constant  Value=KeSMSw6SAcsEntrySecRwLtStCushnFrtUpwdDnwdPosMax_Val
  PA_KeSMSw6SAcsEntrySecRwLtStCushnFrtUpwdDnwdPosMin_Val : Constant  Value=KeSMSw6SAcsEntrySecRwLtStCushnFrtUpwdDnwdPosMin_Val
  PA_KeSMSw6SAcsEntrySecRwLtStCushnFrtUpwdDnwdPos_Val : Constant  Value=KeSMSw6SAcsEntrySecRwLtStCushnFrtUpwdDnwdPos_Val
  PA_KeSMSw6SAcsMd56SecRwLtStCushnFrtUpwdDnwdPosMax_Val : Constant  Value=KeSMSw6SAcsMd56SecRwLtStCushnFrtUpwdDnwdPosMax_Val
  PA_KeSMSw6SAcsMd56SecRwLtStCushnFrtUpwdDnwdPosMin_Val : Constant  Value=KeSMSw6SAcsMd56SecRwLtStCushnFrtUpwdDnwdPosMin_Val
  PA_KeSMSw6SAcsMd56SecRwLtStCushnFrtUpwdDnwdPos_Val : Constant  Value=KeSMSw6SAcsMd56SecRwLtStCushnFrtUpwdDnwdPos_Val
  PA_KeSMSw6SRecoveryMdSecRwLtStCushnFrtUpwdDnwdPosMax_Val : Constant  Value=KeSMSw6SRecoveryMdSecRwLtStCushnFrtUpwdDnwdPosMax_Val
  PA_KeSMSw6SRecoveryMdSecRwLtStCushnFrtUpwdDnwdPosMin_Val : Constant  Value=KeSMSw6SRecoveryMdSecRwLtStCushnFrtUpwdDnwdPosMin_Val
  PA_KeSMSw6SRecoveryMdSecRwLtStCushnFrtUpwdDnwdPos_Val : Constant  Value=KeSMSw6SRecoveryMdSecRwLtStCushnFrtUpwdDnwdPos_Val
  PA_KeSMSwAcsEntrySecRwLtStCushnFrtIUpwdDnwdPosMax_Val : Constant  Value=KeSMSwAcsEntrySecRwLtStCushnFrtIUpwdDnwdPosMax_Val
  PA_KeSMSwAcsEntrySecRwLtStCushnFrtIUpwdDnwdPosMin_Val : Constant  Value=KeSMSwAcsEntrySecRwLtStCushnFrtIUpwdDnwdPosMin_Val
  PA_KeSMSwAcsEntrySecRwLtStCushnFrtIUpwdDnwdPos_Val : Constant  Value=KeSMSwAcsEntrySecRwLtStCushnFrtIUpwdDnwdPos_Val
  PA_KeSMSwAcsMd56SecRwLtStCushnFrtUpwdDnwdPosMax_Val : Constant  Value=KeSMSwAcsMd56SecRwLtStCushnFrtUpwdDnwdPosMax_Val
  PA_KeSMSwAcsMd56SecRwLtStCushnFrtUpwdDnwdPosMin_Val : Constant  Value=KeSMSwAcsMd56SecRwLtStCushnFrtUpwdDnwdPosMin_Val
  PA_KeSMSwAcsMd56SecRwLtStCushnFrtUpwdDnwdPos_Val : Constant  Value=KeSMSwAcsMd56SecRwLtStCushnFrtUpwdDnwdPos_Val
  PA_KeSMSwAcsMd8SecRwLtStCushnFrtUpwdDnwdPosMax_Val : Constant  Value=KeSMSwAcsMd8SecRwLtStCushnFrtUpwdDnwdPosMax_Val
  PA_KeSMSwAcsMd8SecRwLtStCushnFrtUpwdDnwdPosMin_Val : Constant  Value=KeSMSwAcsMd8SecRwLtStCushnFrtUpwdDnwdPosMin_Val
  PA_KeSMSwAcsMd8SecRwLtStCushnFrtUpwdDnwdPos_Val : Constant  Value=KeSMSwAcsMd8SecRwLtStCushnFrtUpwdDnwdPos_Val
  PA_KeSMSwRecoveryMdSecRwLtStCushnFrtUpwdDnwdPosMax_Val : Constant  Value=KeSMSwRecoveryMdSecRwLtStCushnFrtUpwdDnwdPosMax_Val
  PA_KeSMSwRecoveryMdSecRwLtStCushnFrtUpwdDnwdPosMin_Val : Constant  Value=KeSMSwRecoveryMdSecRwLtStCushnFrtUpwdDnwdPosMin_Val
  PA_KeSMSwRecoveryMdSecRwLtStCushnFrtUpwdDnwdPos_Val : Constant  Value=KeSMSwRecoveryMdSecRwLtStCushnFrtUpwdDnwdPos_Val
  TrgtPosSelcNot4sMotor{,1..3} (4 alike) : TrgtPosSelcLib/TrgtPosSelcNo4sMd  SystemSampleTime=-1
  ComfortMdR2LZeroTrgtPosCalib_TrgtPosArray_write : Outport
      settings: EnsureOutportIsVirtual=on
  EZEMdR2LZeroTrgtPosCalib_TrgtPosArray_write : Outport  Port=2
      settings: EnsureOutportIsVirtual=on
  Md8R2LZeroTrgtPosCalib_TrgtPosArray_write : Outport  Port=3
      settings: EnsureOutportIsVirtual=on
  Md56R2LZeroTrgtPosCalib_TrgtPosArray_write : Outport  Port=4
      settings: EnsureOutportIsVirtual=on
  wires:
  [Is6s] -> TrgtPosSelcNot4sMotor2/1
  PA_KeSMSwAcsMd8SecRwLtStCushnFrtUpwdDnwdPos_Val/1 -> TrgtPosSelcNot4sMotor2/5
  PA_KeSMSwRecoveryMdSecRwLtStCushnFrtUpwdDnwdPos_Val/1 -> TrgtPosSelcNot4sMotor/5
  [invalidPos] -> TrgtPosSelcNot4sMotor2/3
  PA_KeSMSw6SAcsEntrySecRwLtStCushnFrtUpwdDnwdPosMax_Val/1 -> TrgtPosSelcNot4sMotor1/3
  PA_KeSMSwAcsEntrySecRwLtStCushnFrtIUpwdDnwdPosMin_Val/1 -> TrgtPosSelcNot4sMotor1/7
  Data Type Conversion2/1 -> Md56R2LZeroTrgtPosCalib_TrgtPosArray_write/1
  Data Type Conversion/1 -> ComfortMdR2LZeroTrgtPosCalib_TrgtPosArray_write/1
  PA_KeSMSwAcsEntrySecRwLtStCushnFrtIUpwdDnwdPosMax_Val/1 -> TrgtPosSelcNot4sMotor1/6
  PA_KeSMSwAcsEntrySecRwLtStCushnFrtIUpwdDnwdPos_Val/1 -> TrgtPosSelcNot4sMotor1/5
  PA_KeSMSw6SAcsEntrySecRwLtStCushnFrtUpwdDnwdPosMin_Val/1 -> TrgtPosSelcNot4sMotor1/4
  PA_KeSMSw6SAcsMd56SecRwLtStCushnFrtUpwdDnwdPos_Val/1 -> TrgtPosSelcNot4sMotor3/2
  TrgtPosSelcNot4sMotor2/1 -> Md8R2LZeroTrgtPosCalib_TrgtPosArray_write/1
  PA_KeSMSw6SAcsEntrySecRwLtStCushnFrtUpwdDnwdPos_Val/1 -> TrgtPosSelcNot4sMotor1/2
  [invalidPos] -> TrgtPosSelcNot4sMotor2/4
  [invalidPos] -> TrgtPosSelcNot4sMotor2/2
  PA_KeSMSwAcsMd8SecRwLtStCushnFrtUpwdDnwdPosMax_Val/1 -> TrgtPosSelcNot4sMotor2/6
  PA_KeSMSwRecoveryMdSecRwLtStCushnFrtUpwdDnwdPosMin_Val/1 -> TrgtPosSelcNot4sMotor/7
  PA_KeSMSwAcsMd8SecRwLtStCushnFrtUpwdDnwdPosMin_Val/1 -> TrgtPosSelcNot4sMotor2/7
  PA_KeSMSwAcsMd56SecRwLtStCushnFrtUpwdDnwdPosMin_Val/1 -> TrgtPosSelcNot4sMotor3/7
  StNumFlg_Is6s_read/1 -> [Is6s], TrgtPosSelcNot4sMotor1/1, TrgtPosSelcNot4sMotor/1
  TrgtPosSelcNot4sMotor1/1 -> Data Type Conversion1/1
  PA_KeSMSw6SRecoveryMdSecRwLtStCushnFrtUpwdDnwdPosMax_Val/1 -> TrgtPosSelcNot4sMotor/3
  TrgtPosSelcNot4sMotor/1 -> Data Type Conversion/1
  Data Type Conversion1/1 -> EZEMdR2LZeroTrgtPosCalib_TrgtPosArray_write/1
  PA_KeSMSwRecoveryMdSecRwLtStCushnFrtUpwdDnwdPosMax_Val/1 -> TrgtPosSelcNot4sMotor/6
  PA_KeSMSw6SRecoveryMdSecRwLtStCushnFrtUpwdDnwdPos_Val/1 -> TrgtPosSelcNot4sMotor/2
  PA_KeSMSw6SRecoveryMdSecRwLtStCushnFrtUpwdDnwdPosMin_Val/1 -> TrgtPosSelcNot4sMotor/4
  [Is6s] -> TrgtPosSelcNot4sMotor3/1
  PA_KeSMSwAcsMd56SecRwLtStCushnFrtUpwdDnwdPosMax_Val/1 -> TrgtPosSelcNot4sMotor3/6
  PA_KeSMSw6SAcsMd56SecRwLtStCushnFrtUpwdDnwdPosMax_Val/1 -> TrgtPosSelcNot4sMotor3/3
  PA_KeSMSwAcsMd56SecRwLtStCushnFrtUpwdDnwdPos_Val/1 -> TrgtPosSelcNot4sMotor3/5
  TrgtPosSelcNot4sMotor3/1 -> Data Type Conversion2/1
  PA_KeSMSw6SAcsMd56SecRwLtStCushnFrtUpwdDnwdPosMin_Val/1 -> TrgtPosSelcNot4sMotor3/4
  Constant/1 -> [invalidPos]
